simulink library "OrionBMS2"  (R2024a)
settings: Solver=VariableStepAuto  StartTime=0.0  StopTime=10.0  RelTol=1e-3
undefined symbols (not defined in the file or in its folder): raptor_xcp_function, StateCAN
libraries: Utilities x17, Raptor_lib x5, simulink x1
settings Model: Creator=serga  LastModifiedBy=serga

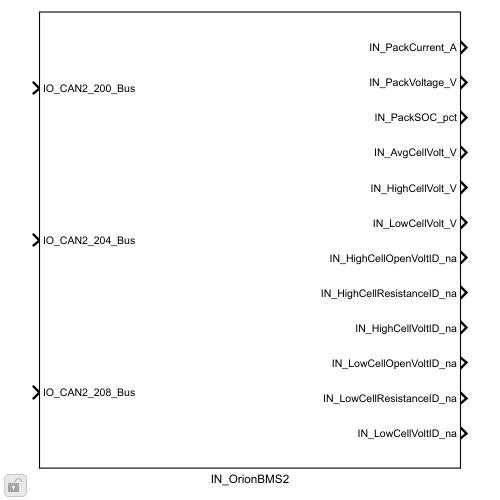
[thumbnail: Simulink's stored preview of the top-level diagram]
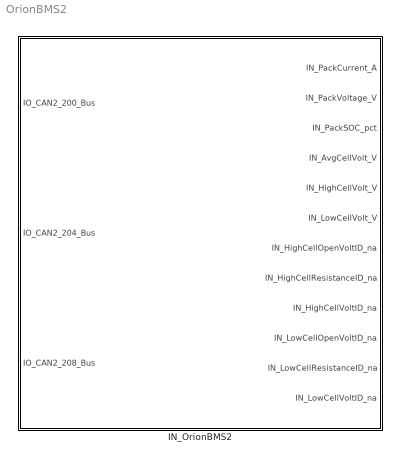
== system OrionBMS2 ==
  IN_OrionBMS2 : Subsystem

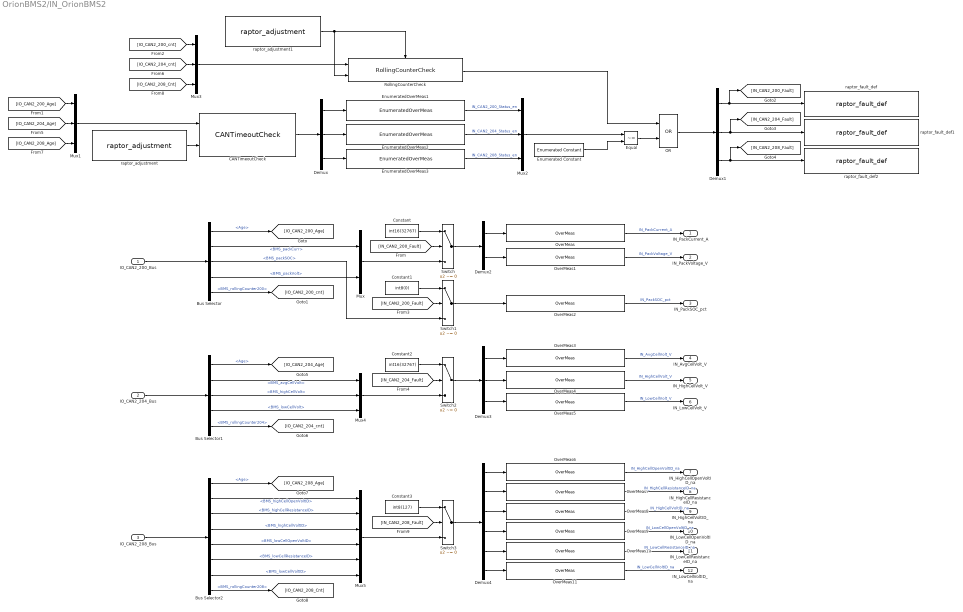
== system OrionBMS2/IN_OrionBMS2 ==
  IO_CAN2_200_Bus : Inport
  IO_CAN2_204_Bus : Inport  Port=2
  IO_CAN2_208_Bus : Inport  Port=3
  Bus Selector : BusSelector  OutputSignals=Age,BMS_packCurr,BMS_packSOC,BMS_packVolt,BMS_rollingCounter200
  Bus Selector1 : BusSelector  OutputSignals=Age,BMS_avgCellVolt,BMS_highCellVolt,BMS_lowCellVolt,BMS_rollingCounter204
  Bus Selector2 : BusSelector  OutputSignals=Age,BMS_highCellOpenVoltID,BMS_highCellResistanceID,BMS_highCellVoltID,BMS_lowCellOpenVoltID,BMS_lowCellResistanceID,BMS_lowCellVoltID,BMS_rollingCounter208
  CANTimeoutCheck : Utilities/CANTimeoutCheck
  Constant : Constant  Value=int16(32767)
  Constant1 : Constant  Value=int8(0)
  Constant2 : Constant  Value=int16(32767)
  Constant3 : Constant  Value=int8(127)
  Demux : Demux  Outputs=3
  Demux1 : Demux  Outputs=3
  Demux2 : Demux  Outputs=2
  Demux3 : Demux  Outputs=3
  Demux4 : Demux  Outputs=6
  Enumerated Constant : simulink/Sources/Enumerated Constant  OutDataTypeStr=Enum: StateCAN  Value=StateCAN.Normal  SampleTime=inf
  EnumeratedOverMeas1 : Utilities/EnumeratedOverMeas  sigName='IN_CAN2_200_Status_en'  enumName='StateCAN'
  EnumeratedOverMeas2 : Utilities/EnumeratedOverMeas  sigName='IN_CAN2_204_Status_en'  enumName='StateCAN'
  EnumeratedOverMeas3 : Utilities/EnumeratedOverMeas  sigName='IN_CAN2_208_Status_en'  enumName='StateCAN'
  Equal : RelationalOperator  Operator=~=  OutDataTypeStr=boolean  RndMeth=Simplest  InputSameDT=off
  Mux : Mux  Inputs=2
  Mux{1..4} (4 alike) : Mux  Inputs=3
  Mux5 : Mux  Inputs=6
  OR : Logic  Operator=OR  AllPortsSameDT=off  OutDataTypeStr=boolean
  OverMeas : Utilities/OverMeas  sigName='IN_PackCurrent_A'  minimum=-inf  maximum=inf
  OverMeas1 : Utilities/OverMeas  sigName='IN_PackVoltage_V'  minimum=-inf  maximum=inf
  OverMeas10 : Utilities/OverMeas  sigName='IN_LowCellResistanceID_na'  minimum=-inf  maximum=inf
  OverMeas11 : Utilities/OverMeas  sigName='IN_LowCellVoltID_na'  minimum=-inf  maximum=inf
  OverMeas2 : Utilities/OverMeas  sigName='IN_PackSOC_pct'  minimum=-inf  maximum=inf
  OverMeas3 : Utilities/OverMeas  sigName='IN_AvgCellVolt_V'  minimum=-inf  maximum=inf
  OverMeas4 : Utilities/OverMeas  sigName='IN_HighCellVolt_V'  minimum=-inf  maximum=inf
  OverMeas5 : Utilities/OverMeas  sigName='IN_LowCellVolt_V'  minimum=-inf  maximum=inf
  OverMeas6 : Utilities/OverMeas  sigName='IN_HighCellOpenVoltID_na'  minimum=-inf  maximum=inf
  OverMeas7 : Utilities/OverMeas  sigName='IN_HighCellResistanceID_na'  minimum=-inf  maximum=inf
  OverMeas8 : Utilities/OverMeas  sigName='IN_HighCellVoltID_na'  minimum=-inf  maximum=inf
  OverMeas9 : Utilities/OverMeas  sigName='IN_LowCellOpenVoltID_na'  minimum=-inf  maximum=inf
  RollingCounterCheck : Utilities/RollingCounterCheck
  Switch{,1..3} (4 alike) : Switch  Criteria=u2 ~= 0  SaturateOnIntegerOverflow=off  InputSameDT=off
  raptor_adjustment : Raptor_lib/Data Storage/raptor_adjustment  paramName='IN_OrionBMS2TOThresh_na'  nameSource=Parameter  initValue=200  dataType=uint32  storage=Calibration  calDispType=Number  calEnum={'False', 'True'}  calGain=1.0  calOffset=0.0  calMax=inf  calMin=-inf  calFormat='-1'  calUnit=''  calHelp=''  calAccess=1  calFunction=raptor_xcp_function(gcb)  calDispHeaders=off  calColHeaders={'Col1' 'Col2' 'Col3'}  calRowHeaders={'Row1' 'Row2' 'Row3'}
      settings: SourceProductName=Raptor
  raptor_adjustment1 : Raptor_lib/Data Storage/raptor_adjustment  paramName='IN_OrionBMS2RollingCounterEnable_bool'  nameSource=Parameter  initValue=1  dataType=boolean  storage=Calibration  calDispType=Number  calEnum={'False', 'True'}  calGain=1.0  calOffset=0.0  calMax=inf  calMin=-inf  calFormat='-1'  calUnit=''  calHelp=''  calAccess=1  calFunction=raptor_xcp_function(gcb)  calDispHeaders=off  calColHeaders={'Col1' 'Col2' 'Col3'}  calRowHeaders={'Row1' 'Row2' 'Row3'}
      settings: SourceProductName=Raptor
  raptor_fault_def : Raptor_lib/Faults/raptor_fault_def  faultName='IN_CAN2_200_Fault'  persist=on  sticky=off  emisRelated=off  singleTrip=off  clearMethod=Standard  xLimit=25  yLimit=50  calEnable=on  addDisable=off  calAccess=1  calFunction='System | FaultManager'
      settings: SourceProductName=Raptor
  raptor_fault_def1 : Raptor_lib/Faults/raptor_fault_def  faultName='IN_CAN2_204_Fault'  persist=on  sticky=off  emisRelated=off  singleTrip=off  clearMethod=Standard  xLimit=25  yLimit=50  calEnable=on  addDisable=off  calAccess=1  calFunction='System | FaultManager'
      settings: SourceProductName=Raptor
  raptor_fault_def2 : Raptor_lib/Faults/raptor_fault_def  faultName='IN_CAN2_208_Fault'  persist=on  sticky=off  emisRelated=off  singleTrip=off  clearMethod=Standard  xLimit=25  yLimit=50  calEnable=on  addDisable=off  calAccess=1  calFunction='System | FaultManager'
      settings: SourceProductName=Raptor
  IN_PackCurrent_A : Outport
  IN_PackVoltage_V : Outport  Port=2
  IN_PackSOC_pct : Outport  Port=3
  IN_AvgCellVolt_V : Outport  Port=4
  IN_HighCellVolt_V : Outport  Port=5
  IN_LowCellVolt_V : Outport  Port=6
  IN_HighCellOpenVoltID_na : Outport  Port=7
  IN_HighCellResistanceID_na : Outport  Port=8
  IN_HighCellVoltID_na : Outport  Port=9
  IN_LowCellOpenVoltID_na : Outport  Port=10
  IN_LowCellResistanceID_na : Outport  Port=11
  IN_LowCellVoltID_na : Outport  Port=12
  wires:
  OverMeas11/1 -> IN_LowCellVoltID_na/1  "IN_LowCellVoltID_na"
  OverMeas10/1 -> IN_LowCellResistanceID_na/1  "IN_LowCellResistanceID_na"
  OverMeas9/1 -> IN_LowCellOpenVoltID_na/1  "IN_LowCellOpenVoltID_na"
  OverMeas8/1 -> IN_HighCellVoltID_na/1  "IN_HighCellVoltID_na"
  OverMeas7/1 -> IN_HighCellResistanceID_na/1  "IN_HighCellResistanceID_na"
  OverMeas6/1 -> IN_HighCellOpenVoltID_na/1  "IN_HighCellOpenVoltID_na"
  OverMeas5/1 -> IN_LowCellVolt_V/1  "IN_LowCellVolt_V"
  OverMeas4/1 -> IN_HighCellVolt_V/1  "IN_HighCellVolt_V"
  OverMeas3/1 -> IN_AvgCellVolt_V/1  "IN_AvgCellVolt_V"
  OverMeas2/1 -> IN_PackSOC_pct/1  "IN_PackSOC_pct"
  OverMeas1/1 -> IN_PackVoltage_V/1  "IN_PackVoltage_V"
  OverMeas/1 -> IN_PackCurrent_A/1  "IN_PackCurrent_A"
  Demux4/6 -> OverMeas11/1
  Demux4/5 -> OverMeas10/1
  Demux4/4 -> OverMeas9/1
  Demux4/3 -> OverMeas8/1
  Demux4/2 -> OverMeas7/1
  Demux4/1 -> OverMeas6/1
  Switch3/1 -> Demux4/1
  Constant3/1 -> Switch3/1
  [IN_CAN2_208_Fault] -> Switch3/2
  Mux5/1 -> Switch3/3
  [IO_CAN2_208_Cnt] -> Mux3/3
  [IO_CAN2_208_Age] -> Mux1/3
  Bus Selector2/8 -> [IO_CAN2_208_Cnt]  "<BMS_rollingCounter208>"
  Bus Selector2/7 -> Mux5/6  "<BMS_lowCellVoltID>"
  Bus Selector2/6 -> Mux5/5  "<BMS_lowCellResistanceID>"
  Bus Selector2/5 -> Mux5/4  "<BMS_lowCellOpenVoltID>"
  Bus Selector2/4 -> Mux5/3  "<BMS_highCellVoltID>"
  Bus Selector2/3 -> Mux5/2  "<BMS_highCellResistanceID>"
  Bus Selector2/2 -> Mux5/1  "<BMS_highCellOpenVoltID>"
  Bus Selector2/1 -> [IO_CAN2_208_Age]  "<Age>"
  IO_CAN2_208_Bus/1 -> Bus Selector2/1
  [IO_CAN2_204_cnt] -> Mux3/2
  [IO_CAN2_204_Age] -> Mux1/2
  Demux3/3 -> OverMeas5/1
  Demux3/2 -> OverMeas4/1
  Demux3/1 -> OverMeas3/1
  Switch2/1 -> Demux3/1
  Constant2/1 -> Switch2/1
  [IN_CAN2_204_Fault] -> Switch2/2
  Mux4/1 -> Switch2/3
  Bus Selector1/5 -> [IO_CAN2_204_cnt]  "<BMS_rollingCounter204>"
  Bus Selector1/4 -> Mux4/3  "<BMS_lowCellVolt>"
  Bus Selector1/3 -> Mux4/2  "<BMS_highCellVolt>"
  Bus Selector1/2 -> Mux4/1  "<BMS_avgCellVolt>"
  Bus Selector1/1 -> [IO_CAN2_204_Age]  "<Age>"
  IO_CAN2_204_Bus/1 -> Bus Selector1/1
  Switch1/1 -> OverMeas2/1
  [IN_CAN2_200_Fault] -> Switch1/2
  Constant1/1 -> Switch1/1
  Demux2/2 -> OverMeas1/1
  Demux2/1 -> OverMeas/1
  Switch/1 -> Demux2/1
  Demux1/3 -> raptor_fault_def2/1, [IN_CAN2_208_Fault]
  Demux1/2 -> raptor_fault_def1/1, [IN_CAN2_204_Fault]
  Demux1/1 -> [IN_CAN2_200_Fault], raptor_fault_def/1
  OR/1 -> Demux1/1
  [IO_CAN2_200_cnt] -> Mux3/1
  Mux3/1 -> RollingCounterCheck/1
  RollingCounterCheck/1 -> OR/1
  raptor_adjustment1/1 -> RollingCounterCheck/Enable, RollingCounterCheck/2
  Equal/1 -> OR/2
  Mux2/1 -> Equal/1
  Enumerated Constant/1 -> Equal/2
  EnumeratedOverMeas3/1 -> Mux2/3  "IN_CAN2_208_Status_en"
  EnumeratedOverMeas2/1 -> Mux2/2  "IN_CAN2_204_Status_en"
  EnumeratedOverMeas1/1 -> Mux2/1  "IN_CAN2_200_Status_en"
  Demux/3 -> EnumeratedOverMeas3/1
  Demux/2 -> EnumeratedOverMeas2/1
  Demux/1 -> EnumeratedOverMeas1/1
  CANTimeoutCheck/1 -> Demux/1
  raptor_adjustment/1 -> CANTimeoutCheck/2
  [IO_CAN2_200_Age] -> Mux1/1
  Mux1/1 -> CANTimeoutCheck/1
  [IN_CAN2_200_Fault] -> Switch/2
  Constant/1 -> Switch/1
  Mux/1 -> Switch/3
  Bus Selector/5 -> [IO_CAN2_200_cnt]  "<BMS_rollingCounter200>"
  Bus Selector/4 -> Mux/2  "<BMS_packVolt>"
  Bus Selector/3 -> Switch1/3  "<BMS_packSOC>"
  Bus Selector/2 -> Mux/1  "<BMS_packCurr>"
  Bus Selector/1 -> [IO_CAN2_200_Age]  "<Age>"
  IO_CAN2_200_Bus/1 -> Bus Selector/1
